simulink model "QD2_DroneStack_PID_2021a"  (R2026a)
settings: Solver=ode1  StopTime=inf  FixedStep=1/1000  EnableMultiTasking=on
InitFcn:
  | Motor_Mapping_7_Inch
model workspace (MAT data in the model file):
  target_system = 1
undefined symbols (not defined in the file): _Commander, _Stabilizer, datetime, HIL, KT, lf, log_, log_QD2_, m, Motor_Matrix, n, qc_get_step_size, s, saved_data
libraries: quarc_library x106, simulink x24, simulink_extras x3, sl_discontinuities x2
(part 2 of 5)

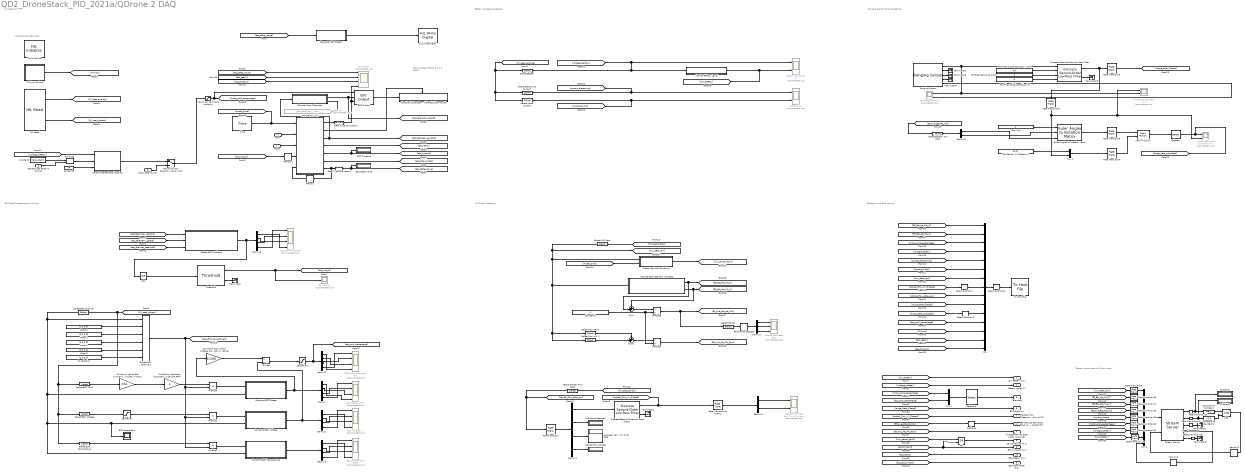
== system QD2_DroneStack_PID_2021a/QDrone 2 DAQ ==
  note: Battery Voltage Processing
  note: IMU Data Processing
  note: ESC Data Processing and Writing
  note: Initialize and read data
  note: Ranging Sensor Data Processing
  note: ESC Numbers
      |
      | FRONT
      | 3 1
      |
      | 2 0
      | BACK
  note: Blackbox and data routing
  note: HIL Read Write
  note: Stream drone data to Python class
  estop : Inport
  "Generalized Force (N, Nm) [4]" : Inport  Port=2
  Motor CMD (%) [4] : Inport  Port=3
  arm : Inport  Port=4
  AND : Logic  IconShape=distinctive  AllPortsSameDT=off  OutDataTypeStr=boolean
  Attitude Estimate from IMU Data : Subsystem
  Attitude Estimates (deg) : Scope  Commented=on  NumInputPorts=3
      settings: Title=Roll Estimates (deg)  ActiveDisplayYMinimum=-29.47666  ActiveDisplayYMaximum=31.43341  DataLoggingVariableName=ScopeData4
  "Average, Max, Min Pixel Rate" : Display
  Battery Monitoring (V) : Scope  Commented=on  NumInputPorts=2
      settings: Title=Battery Level (V)  ActiveDisplayYMinimum=16.17703  ActiveDisplayYMaximum=16.49829  DataLoggingVariableName=ScopeData2
  Choose Motor Telemetry : Subsystem
  Compare To Constant : simulink/Logic and Bit Operations/Compare To Constant  relop===  const=2  OutDataTypeStr=boolean
  Compare To Constant1 : simulink/Logic and Bit Operations/Compare To Constant  relop=>=  const=0  OutDataTypeStr=boolean
  Constant1 : Constant  Value=2
  Constant2 : Constant  Value=Motor_Matrix  OutDataTypeStr=double
  Constant3 : Constant  Value=KT  OutDataTypeStr=double
  Construct ESC Speed : Subsystem
  Construct ESC Temperature : Subsystem
  Construct ESC Voltage : Subsystem
  Convert to equivalent voltage (based on motor Kv rating) : Gain  Gain=1/1300
  Currents (A) : Scope  Commented=on  NumInputPorts=2
      settings: Title=Electronics Current (A)  ActiveDisplayYMinimum=0.11707  ActiveDisplayYMaximum=0.66845  DataLoggingVariableName=ScopeData3
  Data Type Conversion : DataTypeConversion  OutDataTypeStr=uint32  SaturateOnIntegerOverflow=off  RndMeth=Floor
  Data Type Conversion1 : DataTypeConversion  SaturateOnIntegerOverflow=off  RndMeth=Floor
  Demux{,1..3,8} (5 alike) : Demux
  Demux4 : Demux  Outputs=[2 1 3 1]
  Demux5 : Demux  Outputs=2
  Demux6 : Demux  Outputs=2
  Demux7 : Demux  Outputs=3
  Detect ESC Problems : Subsystem
  Discrete Second-Order Low-Pass Filter : quarc_library/Discrete/Discrete Second-Order Low-Pass Filter  params_source=External (input ports)  input_width=1  input_zeta=1  input_init=0  sample_time=qc_get_step_size*ceil(1/25/qc_get_step_size)
      settings: SourceProductName=QUARC Targets
  Discrete Second-Order Low-Pass Filter1 : quarc_library/Discrete/Discrete Second-Order Low-Pass Filter  params_source=Internal (dialog parameters)  input_width=1  input_zeta=1  input_init=0  sample_time=0.01
      settings: SourceProductName=QUARC Targets
  Display5 : Display
  Display6 : Display
  Divide : Product  Inputs=*/
  Divide by half of the number of poles in motor : Gain  Gain=2/14
  ESC Comm Problem : Scope  Commented=on  NumInputPorts=4
      settings: Title=Front Left (Motor 3)  ActiveDisplayYMinimum=-0.125  ActiveDisplayYMaximum=1.125  DataLoggingVariableName=ScopeData6
  ESC Motor Command (%) : Scope  Commented=on  NumInputPorts=4
      settings: Title=Front Left (Motor 3)  ActiveDisplayYMinimum=-0.00954  ActiveDisplayYMaximum=0.0859
  ESC Not OK : Scope  Commented=on
      settings: ActiveDisplayYMinimum=-0.125  ActiveDisplayYMaximum=1.125
  ESC Output : quarc_library/Data Acquisition/Generic/Transformations/ESC Output  protocol=DShot (raw)  sign=Unsigned
      settings: AttributesFormatString=%<protocol>  SourceProductName=QUARC Targets
  ESC Select Raw : Scope
      settings: ActiveDisplayYMinimum=-0.375  ActiveDisplayYMaximum=3.375  DataLoggingVariableName=ScopeData5
  ESC Speed (RPM) : Scope  Commented=on  NumInputPorts=4
      settings: Title=Front Left (Motor 3)  ActiveDisplayYMinimum=651.78571  ActiveDisplayYMaximum=1705.35714  DataLoggingVariableName=ScopeData4
  ESC State Value : Display
  ESC States : Scope  Commented=on  NumInputPorts=4
      settings: Title=ESC State  ActiveDisplayYMinimum=-11  ActiveDisplayYMaximum=99
  ESC Temperature (degC) : Scope  Commented=on  NumInputPorts=4
      settings: Title=Front Left (Motor 3)  ActiveDisplayYMinimum=-5.125  ActiveDisplayYMaximum=46.125  DataLoggingVariableName=ScopeData2
  ESC Timeout : Display
  ESC Voltage (V) : Scope  Commented=on  NumInputPorts=4
      settings: Title=Front Left (Motor 3)  ActiveDisplayYMinimum=-2.115  ActiveDisplayYMaximum=19.035  DataLoggingVariableName=ScopeData8
  Enabled Subsystem - Write ESC Commands : Subsystem  TreatAsAtomicUnit=on
  Euler Angles to Rotation Matrix : quarc_library/Math Operations/Matrices/Euler Angles to Rotation Matrix  menu_order=Relative Z-Y-X
      settings: SourceProductName=QUARC Targets
  Extract ESC Channels : MultiPortSwitch  DataPortOrder=Zero-based contiguous  Inputs=4  DataPortForDefault=Additional data port  zeroidx=on  SaturateOnIntegerOverflow=off  InputSameDT=off
  Force to percentage Mapping : MATLAB Function  TreatAsAtomicUnit=on
  Generate LED Pattern : Subsystem
  Goto19 : Goto  Commented=on  GotoTag=esc_telemetry_index
  HIL Initialize : quarc_library/Data Acquisition/Generic/Configuration/HIL Initialize  object_name=HIL-1  board_type=qdrone2  board_number=0  board_options=gyro0_fs=250;gyro0_rate=500;gyro0_bw=125;gyro0_ord=3;accel0_fs=16;accel0_rate=1000;accel0_bw=250;accel0_ord=3;temp0_bw=4000;gyro1_fs=250;gyro1_rate=500;gyro1_bw=125;gyro1_ord=3;accel1_fs=16;accel1_rate=1000;accel1_bw=400;accel1_ord=3;temp1_bw=4000;enc0_dir=0;enc1_dir=0;pwm03_dshot=1;opt_rate=121;  exclusive=off  active=on  hardware_clocks=[]  clock_modes=[]  initial_clock_frequencies=[]  set_clock_params_at_start=off  set_clock_params_at_switch_in=off  set_clock_frequencies_at_start=off  set_clock_frequencies_at_switch_in=off  analog_input_channels=[0:3]  analog_input_configurations=[]  analog_input_maximums=[3.3]  analog_input_minimums=[0]  set_analog_input_params_at_start=off  set_analog_input_params_at_switch_in=off  analog_output_channels=[]  analog_output_maximums=[]  analog_output_minimums=[]  initial_analog_outputs=[]  final_analog_outputs=[]  watchdog_analog_outputs=[]  set_analog_output_params_at_start=off  set_analog_output_params_at_switch_in=off  set_analog_outputs_at_start=off  set_analog_outputs_at_switch_in=off  set_analog_outputs_at_terminate=off  set_analog_outputs_at_switch_out=off  set_analog_outputs_on_watchdog=off  digital_input_channels=[0:5]  digital_output_channels=[6:11]  digital_output_configuration=[]  initial_digital_outputs=[0]  final_digital_outputs=[0]  watchdog_digital_outputs=[0 0 0 0 0 0]  set_digital_output_params_at_start=off  set_digital_output_params_at_switch_in=off  set_digital_outputs_at_start=on  set_digital_outputs_at_switch_in=off  set_digital_outputs_at_terminate=on  set_digital_outputs_at_switch_out=off  set_digital_outputs_on_watchdog=off  encoder_channels=[0:1]  quadrature=[4]  encoder_filter_frequency=100e6/1  initial_encoder_counts=[0]  set_encoder_params_at_start=on  set_encoder_params_at_switch_in=off  set_encoder_counts_at_start=on  set_encoder_counts_at_switch_in=off  pwm_channels=[0:5]  pwm_modes=[6 6 6 6 0]  pwm_frequency=[600000]  pwm_configuration=[0]  pwm_alignment=[0]  pwm_polarity=[1]  pwm_leading_deadband=[]  pwm_trailing_deadband=[]  initial_pwm_outputs=[0]  final_pwm_outputs=[0]  watchdog_pwm_outputs=[0]  set_pwm_params_at_start=on  set_pwm_params_at_switch_in=off  set_pwm_outputs_at_start=on  set_pwm_outputs_at_switch_in=off  set_pwm_outputs_at_terminate=on  set_pwm_outputs_at_switch_out=off  set_pwm_outputs_on_watchdog=on  other_output_channels=[]  initial_other_outputs=[]  final_other_outputs=[]  watchdog_other_outputs=[]  set_other_outputs_at_start=on  set_other_outputs_at_switch_in=off  set_other_outputs_at_terminate=on  set_other_outputs_at_switch_out=off  set_other_outputs_on_watchdog=off
  HIL Read : quarc_library/Data Acquisition/Generic/Immediate I//O/HIL Read  object_name=HIL-1  analog_channels=[3 1:2]  encoder_channels=[]  digital_channels=[]  other_channels=[3000:3002 4000:4002 3003:3005 4003:4005 17000:17006 17008:17009 17007 17010]  sample_time=qc_get_step_size  active=on  vector_output=on  port_labels=channel numbers  data_type_mode=Inherit via back propagation  encoder_data_type=double  digital_data_type=boolean
  HIL Write Digital : quarc_library/Data Acquisition/Generic/Immediate I//O/HIL Write Digital  object_name=HIL-1  channels=[6:11]  sample_time=-1  active=off  vector_input=on  port_labels=channel numbers
      settings: SourceProductName=QUARC Targets
  Height Estimate Compares (m) : Scope  Commented=on  NumInputPorts=2
      settings: Title=ToF Range Projected (m)  ActiveDisplayYMinimum=-0.10933  ActiveDisplayYMaximum=0.98394  DataLoggingVariableName=ScopeData3
  MATLAB Function : MATLAB Function  TreatAsAtomicUnit=on
  Manual Switch - Select Command Input : ManualSwitch
  Matrix Multiply : Product  Multiplication=Matrix(*)
  "Maximum Command Authority " : Saturate  UpperLimit=[1 1 1 1]  LowerLimit=[1 1 1 1]*0.025
  Memory : Memory
  Memory1 : Memory
  Memory2 : Memory  InheritSampleTime=on
  Memory3 : Memory  InheritSampleTime=on
  Monitor Battery Level : Subsystem
  Motor 0 : Constant  Value=[1 0 0 0]
  Motor 1 : Constant  Value=[0 1 0 0]
  Motor 2 : Constant  Value=[0 0 1 0]
  Motor 3 : Constant  Value=[0 0 0 1]
  Multiple by resolution (supposed to be 100 RPM) : Gain
  Mux : Mux  Inputs=15
  Mux1 : Mux  Inputs=2
  Mux2 : Mux  Inputs=2
  Mux3 : Mux  Inputs=9
  No selection : Constant  Value=[0 0 0 0]
  Number of Features : Display
  OR : Logic  Operator=OR  IconShape=distinctive  AllPortsSameDT=off  OutDataTypeStr=boolean
  OR1 : Logic  Operator=OR  Inputs=1  IconShape=distinctive  AllPortsSameDT=off  OutDataTypeStr=boolean
  Optical Flow Rate (Body Frame) (pixel/s) : Scope  Commented=on  NumInputPorts=2
      settings: Title=Body X Flow Rate (pixel/s)  ActiveDisplayYMinimum=-1312.1789  ActiveDisplayYMaximum=1008.97959
  Optical Flow Shutter : Display
  Product : Product
  Product1 : Product
  Product2 : Product
  Product3 : Product  Inputs=*/
  Product4 : Product  Inputs=*/
  Product5 : Product  Multiplication=Matrix(*)
  Radians to Degrees : simulink_extras/Transformations/Radians to Degrees
  Ranging Sensor : quarc_library/Devices/Third-Party/Sensors/Ranging Sensor  sensor_type=VL53L1X Time-of-flight  uri=i2c-cpu://localhost:0?address='0x29',baud='400000',memsize='512'  ranging_distance=Long  timing_budget=0.033  measurement_period=0.040  output_mode=Fixed-size output  samples_per_revolution=1300  max_distance=0.050  max_angle=5  sample_time=qc_get_step_size*ceil(1/25/qc_get_step_size)  show_versions=off  active=on
      settings: SourceProductName=QUARC Targets
  Rate Transition : RateTransition  OutPortSampleTime=0.01
  Rate Transition to 100Hz : RateTransition  OutPortSampleTime=0.01
  Rate Transition{1..2,7..12,14..20} (15 alike) : RateTransition
  Rate Transition3 : RateTransition  OutPortSampleTime=qc_get_step_size*ceil(1/25/qc_get_step_size)
  Rate Transition4 : RateTransition  OutPortSampleTime=qc_get_step_size*ceil(1/25/qc_get_step_size)
  Rate Transition5 : RateTransition  OutPortSampleTime=qc_get_step_size*ceil(1/25/qc_get_step_size)
  Rate Transition6 : RateTransition  OutPortSampleTime=qc_get_step_size
  Reshape : Reshape
  Saturation : Saturate  UpperLimit=17  LowerLimit=10
  Saturation1 : Saturate  UpperLimit=1  LowerLimit=0
  Select Battery : Selector  InputPortWidth=3  IndexOptions=Index vector (dialog)  Indices=[1]  OutputSizes=1
  Select ESC Channel : Selector  InputPortWidth=23  IndexOptions=Index vector (dialog)  Indices=[22]  OutputSizes=1
  Select ESC RPPM : Selector  InputPortWidth=23  IndexOptions=Index vector (dialog)  Indices=[20]  OutputSizes=1
  Select ESC Temperature : Selector  InputPortWidth=23  IndexOptions=Index vector (dialog)  Indices=[23]  OutputSizes=1
  Select ESC Voltage : Selector  InputPortWidth=23  IndexOptions=Index vector (dialog)  Indices=[21]  OutputSizes=1
  Select Electronics Current : Selector  InputPortWidth=3  IndexOptions=Index vector (dialog)  Indices=[2]  OutputSizes=1
  Select Est Att : Selector  InputPortWidth=9  IndexOptions=Index vector (dialog)  Indices=[1:3]  OutputSizes=1
  Select Est Roll and Pitch : Selector  InputPortWidth=9  IndexOptions=Index vector (dialog)  Indices=[1:2]  OutputSizes=1
  Select IMU Data : Selector  InputPortWidth=23  IndexOptions=Index vector (dialog)  Indices=[1:12]  OutputSizes=1
  Select Motor Current : Selector  InputPortWidth=3  IndexOptions=Index vector (dialog)  Indices=[3]  OutputSizes=1
  Select Optical Flow Data : Selector  InputPortWidth=23  IndexOptions=Index vector (dialog)  Indices=[13:19]  OutputSizes=1
  Select Raw IMU 0 : Selector  InputPortWidth=12  IndexOptions=Index vector (dialog)  Indices=[1:6]  OutputSizes=1
  Select Raw IMU 1 : Selector  InputPortWidth=12  IndexOptions=Index vector (dialog)  Indices=[7:12]  OutputSizes=1
  Selector : Selector  InputPortWidth=3  IndexOptions=Index vector (dialog)  Indices=[3]  OutputSizes=1
  Selector1 : Selector  InputPortWidth=8  IndexOptions=Index vector (dialog)  Indices=[4,8,3,7,2,6,1,5]  OutputSizes=1
  Sensor Failure Monitoring : Subsystem
  Stream Server : quarc_library/Communications/Basic/Stream Server  uri_source=Specify via dialog (do not evaluate)  uri=tcpip://localhost:18491?nagle='off'  send_buffer_size=1460  receive_buffer_size=1460  byte_order=little endian (Intel - LSB first)  optimization=Minimum latency  send_options=Send most recent data  receive_options=Receive most recent data  default_value=0  sample_time=qc_get_step_size*2  active=on  implementation=Use blocking I/O in a separate thread  send_fifo_size=1000  receive_fifo_size=1000  send_priority=0  receive_priority=0  send_dimensions=off  receive_dimensions=off  max_dimensions=-1  data_type=Inherited via back propagation  type_expr=BusObject
      settings: AttributesFormatString="\"tcpip://localhost:18491?nagle='off'\""
  Sum : Sum  Inputs=++|
  Sum1 : Sum  Inputs=++|
  Terminator{,1..7} (8 alike) : Terminator
  Threshold : quarc_library/Discontinuities/Threshold  operator=~=  param_src=Specify via dialog  threshold=0  duration=qc_get_step_size*300
      settings: SourceProductName=QUARC Targets
  Time : quarc_library/Sources/Time/Time  time_source=Wall clock  sample_time=qc_get_step_size
  Timing Monitors : Subsystem
  To Host File : quarc_library/Sinks/To Host/To Host File  source=Specify via dialog (do not evaluate)  file_name=saved_data\%m\log_QD2_%{regexprep(regexprep(char(datetime),':','-'),' ','_')}.mat  variable_name=QD2_data  decimation=1  sample_time=-1  file_format=MAT-file v.4  options=No header or footer  append=off  final_file_name=saved_data\\QD2_DroneStack_PID_2021a\\log_QD2_2026-09-08_13-10-08.mat  encoding=Default  bitrate=2000000
  ToF Filter Cutoff Frequency (rad) : Constant  Value=40
  ToF Filter Damping Ratio : Constant
  ToF Filter Initial Condition (m) : Constant  Value=0
  ToF Range Compare (m) : Scope  Commented=on  NumInputPorts=2
      settings: Title=ToF Range Filtered (m)  ActiveDisplayYMinimum=-0.12994  ActiveDisplayYMaximum=1.16949  DataLoggingVariableName=ScopeData2
  ToF Range Raw (m) : Scope  Commented=on  NumInputPorts=2
      settings: Title=ToF Range (m)  ActiveDisplayYMinimum=0.68027  ActiveDisplayYMaximum=0.99383
  ToF Sensor XY Offsets (m) : Constant  Value=[0 0]
  Zero Yaw : Constant  Value=0
  Low Battery (0,1) : Outport
  Battery Level (V) : Outport  Port=2
  Sensor Failure (0,1) : Outport  Port=3
  "Average BF IMU Data (rad/s, m/s/s) [6]" : Outport  Port=4
  Telemetry : Outport  Port=5
  BF Height (m) : Outport  Port=6
  Optical Flow Measurement (px/s) [2] : Outport  Port=7
  ESC Timeout (0,1) : Outport  Port=8
  ESC Stop Model (0,1) : Outport  Port=9
  ESC Ready (0,1) : Outport  Port=10
  "BF Attitude Estimates (rad, rad/s, rad/s/s) [9]" : Outport  Port=11
  wires:
  Force to percentage Mapping/1(Duty_Cycle) -> Manual Switch - Select Command Input/1
  Motor CMD (%) [4]/1 -> Manual Switch - Select Command Input/2
  "Generalized Force (N, Nm) [4]"/1 -> Product5/2
  [voltage_battery] -> Force to percentage Mapping/1(V_Bat_Act)
  Constant2/1 -> Product5/1
  Manual Switch - Select Command Input/1 -> "Maximum Command Authority "/1
  Constant3/1 -> Force to percentage Mapping/3(KT)
  Product5/1 -> Force to percentage Mapping/2(Motor_Forces)
  Reshape/1 -> "BF Attitude Estimates (rad, rad/s, rad/s/s) [9]"/1
  Saturation1/1 -> Demux2/1, [esc_cmd_percentage]
  [esc_stop_model] -> ESC Stop Model (0,1)/1
  [esc_ready] -> ESC Ready (0,1)/1
  [esc_timeout] -> ESC Timeout (0,1)/1, OR/2
  [BF_Ave_Att_IMU_Raw] -> "Average BF IMU Data (rad/s, m/s/s) [6]"/1
  [imu_sensor_fault] -> OR/1
  [BF_Ave_Est_Att_IMU] -> Reshape/1
  [optical_flow_XY_filtered] -> Optical Flow Measurement (px/s) [2]/1
  [range_data_filtered] -> BF Height (m)/1
  Selector1/1 -> Telemetry/1
  Mux2/1 -> Selector1/1
  [motor_cmd_percentage] -> Mux2/1
  [esc_cmd_percentage] -> Mux2/2
  [voltage_battery] -> Battery Level (V)/1
  [low_battery] -> Low Battery (0,1)/1
  [BF_Est_Att_IMU_1] -> Mux/2
  [voltage_battery] -> Mux/4
  [current_electronics] -> Mux/5
  [optical_flow_XY_filtered] -> Rate Transition7/1
  [esc_cmd_percentage] -> Mux/12
  [BF_Ave_Est_Att_IMU] -> Select Est Roll and Pitch/1
  [esc_ready] -> Mux/14
  [range_data_filtered] -> Mux/10
  Demux6/1 -> Euler Angles to Rotation Matrix/3
  Demux7/1 -> Attitude Estimates (deg)/1
  Ranging Sensor/5 -> ToF Range Raw (m)/2
  Discrete Second-Order Low-Pass Filter/2 -> Terminator5/1
  Radians to Degrees/1 -> Demux7/1
  Demux6/2 -> Euler Angles to Rotation Matrix/2
  Ranging Sensor/4 -> Terminator4/1
  Ranging Sensor/2 -> Terminator2/1
  ToF Filter Cutoff Frequency (rad)/1 -> Discrete Second-Order Low-Pass Filter/2
  ToF Sensor XY Offsets (m)/1 -> Mux1/1
  [Timing] -> Mux/13
  [current_motor] -> Mux/6
  Discrete Second-Order Low-Pass Filter1/1 -> Rate Transition to 100Hz/1, [optical_flow_XY_filtered]
  Demux7/2 -> Attitude Estimates (deg)/2
  Sensor Failure Monitoring/1(Sensor Fault) -> [imu_sensor_fault]
  [esc_state_value] -> Generate LED Pattern/1(ESC States)
  Select Est Att/1 -> Radians to Degrees/1
  Matrix Multiply/1 -> Selector/1
  Select Raw IMU 0/1 -> Sum1/1
  Select Raw IMU 1/1 -> Sum1/2
  [optical_flow_data_raw] -> Mux/9
  [esc_telemetry_select] -> Detect ESC Problems/2(ESC Channel Request [4])
  [esc_ready] -> ESC States/2
  Divide/1 -> Saturation1/1
  Select ESC Voltage/1 -> Saturation/1
  [motor_cmd_percentage] -> Mux/3
  Demux4/4 -> Optical Flow Shutter/1
  Monitor Battery Level/1(Low Battery) -> Battery Monitoring (V)/2, [low_battery]
  Demux3/1 -> ESC Temperature (degC)/4
  Convert to equivalent voltage (based on motor Kv rating)/1 -> Divide/1
  Demux4/2 -> Number of Features/1
  Rate Transition to 100Hz/1 -> Demux5/1
  Mux1/1 -> Rate Transition4/1
  Product3/1 -> [BF_Ave_Est_Att_IMU], Select Est Att/1
  Sum/1 -> Product3/1
  Demux4/1 -> Discrete Second-Order Low-Pass Filter1/1  "Optical Flow Pixel Rate (XY)"
  [imu_data_raw] -> Mux/7
  Demux5/2 -> Optical Flow Rate (Body Frame) (pixel/s)/2
  [esc_state_value] -> ESC States/1
  [hil_read_others] -> Select Optical Flow Data/1
  Discrete Second-Order Low-Pass Filter1/2 -> Terminator1/1
  Demux2/2 -> ESC Motor Command (%)/3
  estop/1 -> MATLAB Function/3(estop)
  Rate Transition4/1 -> Matrix Multiply/2
  Demux7/3 -> Attitude Estimates (deg)/3
  Sum1/1 -> Product4/1
  Threshold/2 -> Terminator/1
  [esc_channel_received] -> Detect ESC Problems/3(ESC Channel Reported [4])
  Generate LED Pattern/1(LED Command) -> HIL Write Digital/1
  Discrete Second-Order Low-Pass Filter/1 -> Rate Transition2/1, Rate Transition5/1
  Memory1/1 -> MATLAB Function/4(esc_problem)
  Demux4/3 -> "Average, Max, Min Pixel Rate"/1
  HIL Read/1 -> [hil_read_analog]
  Memory/1 -> MATLAB Function/5(pre_state)
  Product1/1 -> Construct ESC Voltage/1(ESC Data In [4])
  HIL Read/2 -> [hil_read_others]
  [esc_telemetry_enable] -> Detect ESC Problems/1(ESC Telemetry Enabled)
  Demux1/2 -> ESC Voltage (V)/3
  [model_time] -> Sensor Failure Monitoring/2(Model Time)
  Demux8/4 -> ESC Comm Problem/1
  Euler Angles to Rotation Matrix/1 -> Rate Transition3/1
  Select ESC Temperature/1 -> Product2/1
  MATLAB Function/6(stop_mdl) -> [esc_stop_model]
  Select Motor Current/1 -> Currents (A)/2, [current_motor]
  Construct ESC Voltage/1(ESC Data Out [4]) -> Demux1/1, Divide/2
  Demux1/1 -> ESC Voltage (V)/4
  Construct ESC Temperature/1(ESC Data Out [4]) -> Demux3/1
  Threshold/1 -> [esc_not_ok], ESC Not OK/1
  [esc_timeout] -> Mux/15
  MATLAB Function/4(esc_ready) -> [esc_ready]
  ToF Filter Initial Condition (m)/1 -> Discrete Second-Order Low-Pass Filter/4
  Ranging Sensor/1 -> Discrete Second-Order Low-Pass Filter/1, ToF Range Raw (m)/1, ToF Range Compare (m)/2
  MATLAB Function/2(cmd_enable) -> Enabled Subsystem - Write ESC Commands/Enable
  Ranging Sensor/3 -> Terminator3/1
  Select IMU Data/1 -> Select Raw IMU 1/1, Select Raw IMU 0/1, Attitude Estimate from IMU Data/1(IMU Data [12]), Sensor Failure Monitoring/1(IMU Data [12]), [imu_data_raw]
  No selection/1 -> Extract ESC Channels/6
  [BF_Est_Att_IMU_0] -> Mux/1
  [esc_timeout] -> ESC States/3
  OR1/1 -> Threshold/1
  [hil_read_analog] -> Select Battery/1, Select Motor Current/1, Select Electronics Current/1
  Demux8/2 -> ESC Comm Problem/3
  ToF Filter Damping Ratio/1 -> Discrete Second-Order Low-Pass Filter/3
  MATLAB Function/5(esc_timeout) -> ESC Timeout/1, [esc_timeout]
  Attitude Estimate from IMU Data/2("BF Estimated Attitude for IMU1 (rad, rad/s, rad/2^2) [9]") -> [BF_Est_Att_IMU_1], Sum/1
  Product/1 -> Construct ESC Speed/1(ESC Data In [4])
  [hil_read_others] -> Select IMU Data/1
  Rate Transition5/1 -> Mux1/2, Height Estimate Compares (m)/2, ToF Range Compare (m)/1
  "Maximum Command Authority "/1 -> ESC Output/1, [motor_cmd_percentage]
  Zero Yaw/1 -> Euler Angles to Rotation Matrix/1
  Data Type Conversion/1 -> ESC State Value/1, [esc_state_value]
  Demux1/3 -> ESC Voltage (V)/2
  Demux5/1 -> Optical Flow Rate (Body Frame) (pixel/s)/1
  Saturation/1 -> Product1/1
  Select Optical Flow Data/1 -> Rate Transition/1, [optical_flow_data_raw]
  Demux8/3 -> ESC Comm Problem/2
  Selector/1 -> Height Estimate Compares (m)/1, [range_data_projected]
  Attitude Estimate from IMU Data/1("BF Estimated Attitude for IMU0 (rad, rad/s, rad/2^2) [9]") -> [BF_Est_Att_IMU_0], Sum/2
  Rate Transition/1 -> Demux4/1
  Demux/3 -> ESC Speed (RPM)/2
  Detect ESC Problems/1(ESC Comm Problem [4]) -> Demux8/1, OR1/1
  Demux/4 -> ESC Speed (RPM)/1
  Motor 1/1 -> Extract ESC Channels/3
  Demux2/3 -> ESC Motor Command (%)/2
  Mux/1 -> Rate Transition6/1
  Demux/2 -> ESC Speed (RPM)/3
  Rate Transition3/1 -> Matrix Multiply/1
  Demux/1 -> ESC Speed (RPM)/4
  [esc_not_ok] -> Memory1/1
  Constant1/1 -> Product3/2, Product4/2
  Choose Motor Telemetry/2(Motor telemetry index) -> Goto19/1
  MATLAB Function/3(tele_enable) -> Choose Motor Telemetry/1(enable telemetry), [esc_telemetry_enable]
  [hil_read_others] -> Select ESC Channel/1, Select ESC Voltage/1, Select ESC Temperature/1, Select ESC RPPM/1
  Timing Monitors/1(Timings) -> [Timing]
  Motor 0/1 -> Extract ESC Channels/2
  Demux3/2 -> ESC Temperature (degC)/3
  Select Est Roll and Pitch/1 -> Demux6/1
  Motor 3/1 -> Extract ESC Channels/5
  Product4/1 -> [BF_Ave_Att_IMU_Raw]
  MATLAB Function/1(cmd) -> Data Type Conversion1/1
  Select ESC Channel/1 -> Construct ESC Speed/2(ESC Channel Select), Construct ESC Voltage/2(ESC Channel Select), ESC Select Raw/1, Construct ESC Temperature/2(ESC Channel Select), Extract ESC Channels/1
  Select Electronics Current/1 -> Currents (A)/1, [current_electronics]
  Multiple by resolution (supposed to be 100 RPM)/1 -> Product/1
  Rate Transition1/1 -> Mux/11
  Demux2/1 -> ESC Motor Command (%)/4
  Construct ESC Speed/1(ESC Data Out [4]) -> Convert to equivalent voltage (based on motor Kv rating)/1, Demux/1
  Motor 2/1 -> Extract ESC Channels/4
  Data Type Conversion1/1 -> ESC Output/3, ESC States/4
  MATLAB Function/7(state) -> Memory/1, Data Type Conversion/1
  Rate Transition2/1 -> [range_data_filtered]
  Choose Motor Telemetry/1(Motor telemetry select) -> ESC Output/2, [esc_telemetry_select]
  [range_data_projected] -> Rate Transition1/1
  Time/1 -> MATLAB Function/1(mdl_time), [model_time]
  Extract ESC Channels/1 -> Product2/2, Product1/2, Product/2, [esc_channel_received]
  Select Battery/1 -> Monitor Battery Level/1(Battery (V)), Battery Monitoring (V)/1, [voltage_battery]
  Divide by half of the number of poles in motor/1 -> Multiple by resolution (supposed to be 100 RPM)/1
  Demux1/4 -> ESC Voltage (V)/1
  Demux3/4 -> ESC Temperature (degC)/1
  Demux2/4 -> ESC Motor Command (%)/1
  arm/1 -> MATLAB Function/2(arm)
  ESC Output/1 -> Enabled Subsystem - Write ESC Commands/1(DShot Raw [4])
  Demux3/3 -> ESC Temperature (degC)/2
  Select ESC RPPM/1 -> Divide by half of the number of poles in motor/1
  Demux8/1 -> ESC Comm Problem/4
  Product2/1 -> Construct ESC Temperature/1(ESC Data In [4])
  OR/1 -> Sensor Failure (0,1)/1
  Rate Transition6/1 -> To Host File/1
  Rate Transition7/1 -> Mux/8
  Memory3/1 -> Stream Server/2
  Rate Transition9/1 -> Terminator7/1
  Rate Transition10/1 -> Mux3/6
  Stream Server/1 -> Rate Transition16/1
  Rate Transition17/1 -> Mux3/3
  Rate Transition11/1 -> Mux3/8
  Rate Transition12/1 -> Mux3/7
  [BF_Ave_Est_Att_IMU] -> Rate Transition19/1
  [BF_Est_Att_IMU_0] -> Rate Transition15/1
  AND/1 -> Memory3/1
  Rate Transition20/1 -> Mux3/5
  Rate Transition19/1 -> Mux3/4
  Stream Server/2 -> Rate Transition14/1
  Stream Server/4 -> Memory2/1
  Compare To Constant1/1 -> AND/2
  Memory2/1 -> Mux3/9
  [BF_Est_Att_IMU_1] -> Rate Transition17/1
  [low_battery] -> Rate Transition11/1
  Compare To Constant/1 -> AND/1
  [voltage_battery] -> Rate Transition12/1
  Rate Transition8/1 -> Mux3/1
  [motor_cmd_percentage] -> Rate Transition10/1
  Rate Transition15/1 -> Mux3/2
  [current_motor] -> Rate Transition20/1
  [imu_data_raw] -> Rate Transition8/1
  Stream Server/3 -> Rate Transition9/1
  Rate Transition14/1 -> Display6/1, Compare To Constant1/1
  Rate Transition18/1 -> Terminator6/1  "Connected (bool)"
  Rate Transition16/1 -> Display5/1, Compare To Constant/1
  Stream Server/5 -> Rate Transition18/1
  Mux3/1 -> Stream Server/1

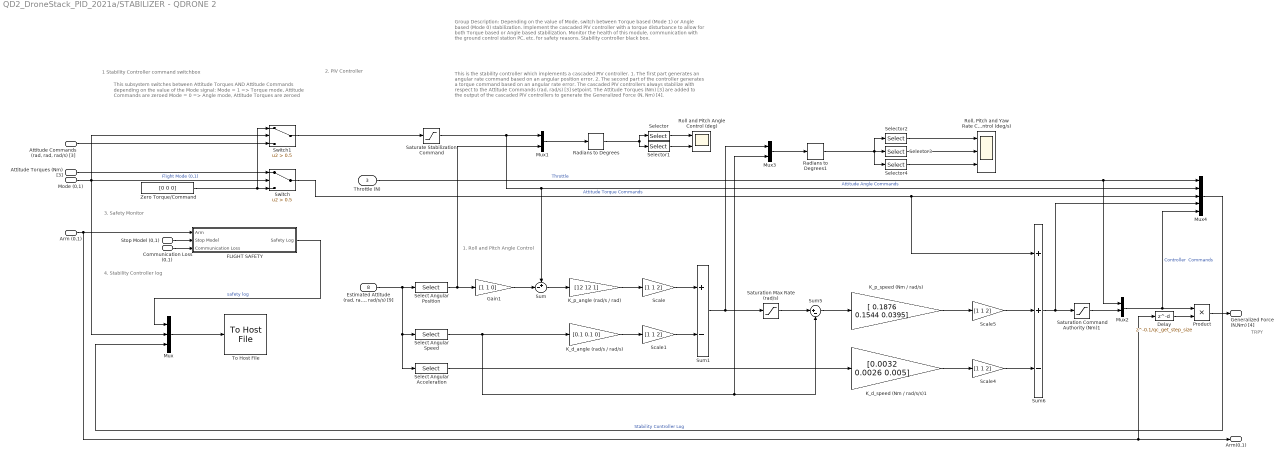
== system QD2_DroneStack_PID_2021a/STABILIZER - QDRONE 2 ==
  note: 3. Safety Monitor
  note: This subsystem switches between Attitude Torques AND Attitude Commands depending on
      | the value of the Mode signal:
      | Mode = 1	=> 		Torque mode, Attitude Commands are zeroed
      | Mode = 0	=> 		Angle mode, Attitude Torques are zeroed
  note: This is the stability controller which implements a cascaded PIV controller.
      | 1. The first part generates an angular rate command based on an angular position error.
      | 2. The second part of the controller generates a torque command based on an angular rate error.
      |
      | The cascaded PIV controllers always stabilize with respect to the Attitude Commands (rad, rad/s) [3] setpoint. The Attitude Torques (Nm) [3] are added to the output of the cascaded PIV controllers to generate the Generalized Force (N, Nm) [4].
  note: 1. Roll and Pitch Angle Control
  note: TRPY
  note: Group Description:
      |
      | Depending on the value of Mode, switch between Torque based (Mode 1) or Angle based (Mode 0) stabilization.
      | Implement the cascaded PIV controller with a torque disturbance to allow for both Torque based or Angle based stabilization.
      | Monitor the health of this module, communication with the ground control station PC, etc. for safety reasons.
      | Stability controller black box.
  note: 1 Stability Controller command switchbox
  note: 4. Stability Controller log
  note: 2. PIV Controller
  Mode (0,1) : Inport
  Stop Model (0,1) : Inport  Port=2
  Throttle (N) : Inport  Port=3
  Attitude Torques (Nm) [3] : Inport  Port=4
  "Attitude Commands (rad, rad, rad/s) [3]" : Inport  Port=5
  Arm (0,1) : Inport  Port=6
  Communication Loss (0,1) : Inport  Port=7
  "Estimated Attitude (rad, rad/s, rad/s/s) [9]" : Inport  Port=8
  Delay : Delay  DelayLength=0.1/qc_get_step_size
  FLIGHT SAFETY : Subsystem
  Gain1 : Gain  Gain=[1 1 0]
  K_d_angle (rad/s / rad/s) : Gain  Gain=[0.1 0.1 0]
  K_d_speed (Nm / rad/s/s)1 : Gain  Gain="[0.0032    0.0026     0.005]"
  K_p_angle (rad/s / rad) : Gain  Gain=[12 12 1]
  K_p_speed (Nm / rad/s) : Gain  Gain="[ 0.1876    0.1544    0.0395]"
  Mux : Mux  Inputs=3
  Mux1 : Mux  Inputs=2
  Mux2 : Mux  Inputs=2
  Mux3 : Mux  Inputs=2
  Mux4 : Mux  Inputs=5
  Product : Product
  Radians to Degrees : simulink_extras/Transformations/Radians to Degrees
  Radians to Degrees1 : simulink_extras/Transformations/Radians to Degrees
  Roll and Pitch Angle Control (deg) : Scope  NumInputPorts=2
      settings: Title=Roll (deg)  ActiveDisplayYMinimum=-2.00555  ActiveDisplayYMaximum=1.8629
  "Roll, Pitch and Yaw Rate Control (deg/s)" : Scope  NumInputPorts=3
      settings: ActiveDisplayYMinimum=-624.0016  ActiveDisplayYMaximum=680.10155  DataLoggingVariableName=ScopeData2
  Saturate Stabilization Command : Saturate  UpperLimit=[pi/4 pi/4 10*pi/18]  LowerLimit=[-pi/4 -pi/4 -10*pi/18]
  Saturation Command Authority (Nm)1 : Saturate  UpperLimit=[1.0915 0.8984 0.0984]  LowerLimit=-[1.0915 0.8984 0.0984]
  Saturation Max Rate (rad/s) : Saturate  UpperLimit=10*pi/3*[1 1 1]  LowerLimit=-10*pi/3*[1 1 1]
  Scale{,1,4..5} (4 alike) : Gain  Gain=[1 1 2]
  Select Angular Acceleration : Selector  InputPortWidth=9  IndexOptions=Index vector (dialog)  Indices=[7:9]  OutputSizes=1
  Select Angular Speed : Selector  InputPortWidth=9  IndexOptions=Index vector (dialog)  Indices=[4:6]  OutputSizes=1
  Select Angular Position : Selector  InputPortWidth=9  IndexOptions=Index vector (dialog)  Indices=[1:3]  OutputSizes=1
  Selector : Selector  InputPortWidth=6  IndexOptions=Index vector (dialog)  Indices=[1 4]  OutputSizes=1
  Selector1 : Selector  InputPortWidth=6  IndexOptions=Index vector (dialog)  Indices=[2 5]  OutputSizes=1
  Selector2 : Selector  InputPortWidth=6  IndexOptions=Index vector (dialog)  Indices=[1 4]  OutputSizes=1
  Selector3 : Selector  InputPortWidth=6  IndexOptions=Index vector (dialog)  Indices=[2 5]  OutputSizes=1
  Selector4 : Selector  InputPortWidth=6  IndexOptions=Index vector (dialog)  Indices=[3 6]  OutputSizes=1
  Sum : Sum  Inputs=+-|
  Sum1 : Sum  Inputs=+-
  Sum5 : Sum  Inputs=|+-
  Sum6 : Sum  Inputs=++-
  Switch : Switch  Criteria=u2 > Threshold  Threshold=0.5  SaturateOnIntegerOverflow=off  InputSameDT=off
  Switch1 : Switch  Criteria=u2 > Threshold  Threshold=0.5  SaturateOnIntegerOverflow=off  InputSameDT=off
  To Host File : quarc_library/Sinks/To Host/To Host File  source=Specify via dialog (do not evaluate)  file_name=saved_data/%m/log_%{regexprep(char(datetime),' ','_')}_Stabilizer.mat  variable_name=stabilizer_data  decimation=1  sample_time=-1  file_format=MAT-file v.5  options=No header or footer  append=off  final_file_name=saved_data/QD2_DroneStack_PID_2021a/log_2026-09-08_13-10-08_Stabilizer.mat  encoding=Default  bitrate=2000000
  Zero Torque/Command : Constant  Value=[0 0 0]
  Generalized Force (N,Nm) [4] : Outport  VectorParamsAs1DForOutWhenUnconnected=off
  Arm(0,1) : Outport  Port=2  VectorParamsAs1DForOutWhenUnconnected=off
  wires:
  Scale1/1 -> Sum1/2
  Scale/1 -> Sum1/1
  Delay/1 -> Product/2
  Zero Torque/Command/1 -> Switch1/1, Switch/3
  Attitude Torques (Nm) [3]/1 -> Switch/1
  "Attitude Commands (rad, rad, rad/s) [3]"/1 -> Switch1/3
  Radians to Degrees/1 -> Selector1/1, Selector/1
  K_d_angle (rad/s / rad/s)/1 -> Scale1/1
  Selector2/1 -> "Roll, Pitch and Yaw Rate Control (deg/s)"/1
  Selector/1 -> Roll and Pitch Angle Control (deg)/1
  Select Angular Speed/1 -> Mux3/2, Sum5/2, K_d_angle (rad/s / rad/s)/1
  K_p_angle (rad/s / rad)/1 -> Scale/1
  Selector4/1 -> "Roll, Pitch and Yaw Rate Control (deg/s)"/3
  Switch1/1 -> Saturate Stabilization Command/1
  Gain1/1 -> Sum/2
  Selector3/1 -> "Roll, Pitch and Yaw Rate Control (deg/s)"/2
  Mux1/1 -> Radians to Degrees/1
  "Estimated Attitude (rad, rad/s, rad/s/s) [9]"/1 -> Select Angular Speed/1, Select Angular Acceleration/1, Select Angular Position/1
  Radians to Degrees1/1 -> Selector3/1, Selector4/1, Selector2/1
  Switch/1 -> Sum6/1, Mux4/3  "Attitude Torque Commands"
  Selector1/1 -> Roll and Pitch Angle Control (deg)/2
  Throttle (N)/1 -> Mux4/1, Mux2/1  "Throttle"
  Select Angular Position/1 -> Mux1/2, Gain1/1
  Mux2/1 -> Product/1, Mux4/5  "Controller  Commands"
  Saturate Stabilization Command/1 -> Mux4/2, Sum/1, Mux1/1  "Attitude Angle Commands"
  Sum1/1 -> Mux3/1, Saturation Max Rate (rad/s)/1
  Mux3/1 -> Radians to Degrees1/1
  Arm (0,1)/1 -> FLIGHT SAFETY/1(Arm), Delay/1, Arm(0,1)/1
  Sum/1 -> K_p_angle (rad/s / rad)/1
  FLIGHT SAFETY/1(Safety Log) -> Mux/1  "safety log"
  Mode (0,1)/1 -> Mux/2, Switch1/2, Switch/2  "Flight Mode (0,1)"
  Mux4/1 -> Mux/3  "Stability Controller Log"
  Mux/1 -> To Host File/1
  Communication Loss (0,1)/1 -> FLIGHT SAFETY/3(Communication Loss)
  Stop Model (0,1)/1 -> FLIGHT SAFETY/2(Stop Model)
  Product/1 -> Generalized Force (N,Nm) [4]/1
  Saturation Max Rate (rad/s)/1 -> Sum5/1
  Sum5/1 -> K_p_speed (Nm / rad/s)/1
  K_p_speed (Nm / rad/s)/1 -> Scale5/1
  K_d_speed (Nm / rad/s/s)1/1 -> Scale4/1
  Scale4/1 -> Sum6/3
  Select Angular Acceleration/1 -> K_d_speed (Nm / rad/s/s)1/1
  Sum6/1 -> Mux4/4, Saturation Command Authority (Nm)1/1
  Saturation Command Authority (Nm)1/1 -> Mux2/2
  Scale5/1 -> Sum6/2

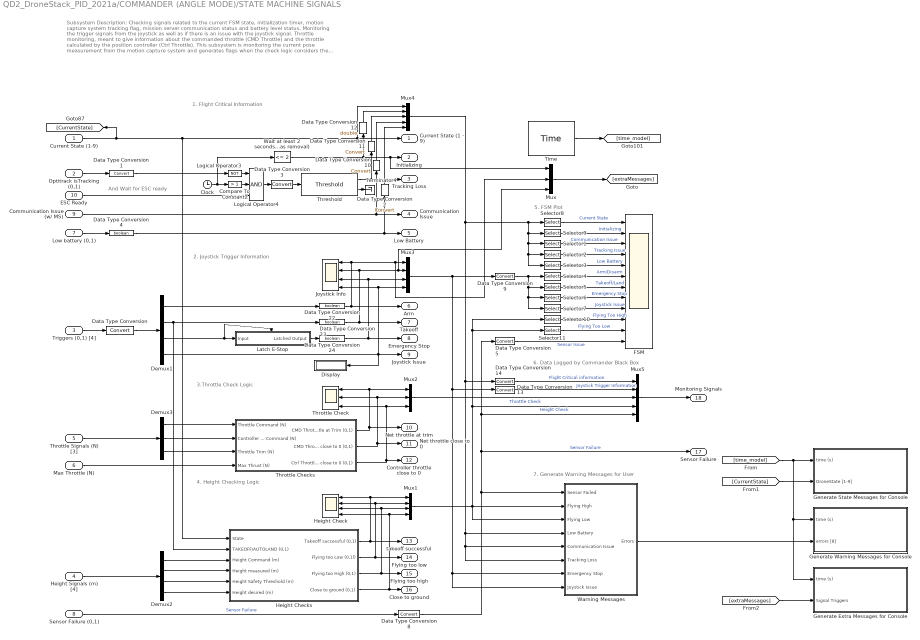
== system QD2_DroneStack_PID_2021a/COMMANDER (ANGLE MODE)/STATE MACHINE SIGNALS ==
  note: 4. Height Checking Logic
  note: 3.Throttle Check Logic
  note: 2. Joystick Trigger Information
  note: 1. Flight Critical Information
  note: 6. Data Logged by Commander Black Box
  note: 5. FSM Plot
  note: 7. Generate Warning Messages for User
  note: Subsystem Description:
      | Checking signals related to the current FSM state, initialization timer, motion capture system tracking flag, mission server communication status and battery level status.
      | Monitoring the trigger signals from the joystick as well as if there is an issue with the joystick signal.
      | Throttle monitoring, meant to give information about the commanded throttle (CMD Throttle) and the throttle calculated by the position controller (Ctrl Throttle).
      | This subsystem is monitoring the current pose measurement from the motion capture system and generates flags when the check logic considers the QDrone flying to close to ground, too high or too low as well as generate a successful take off flag.
      | A subset of the FSM monitoring signals are shown using this scope. These signals are what Quanser considers importnat for flight.
      | FSM signals sent to the blackbox for post flight monitoring.
      | Error message generation based on flags generated by the FSM signal checks.
  note: And Wait for ESC ready
  Current State (1-9) : Inport
  "Optitrack isTracking (0,1)  " : Inport  Port=2
  Triggers (0,1) [4] : Inport  Port=3
  Height Signals (m) [4] : Inport  Port=4
  Throttle Signals (N) [3] : Inport  Port=5
  "Max Throttle (N) " : Inport  Port=6
  Low battery (0,1) : Inport  Port=7
  Sensor Failure (0,1) : Inport  Port=8
  Communication Issue (w/ MS) : Inport  Port=9
  ESC Ready : Inport  Port=10
  Clock : Clock
  Compare To Constant2 : simulink/Logic and Bit Operations/Compare To Constant  relop=>  const=1  OutDataTypeStr=boolean
  Data Type Conversion{,1..3,5,8..11,13..14} (11 alike) : DataTypeConversion  SaturateOnIntegerOverflow=off  RndMeth=Floor
  Data Type Conversion12 : DataTypeConversion  OutDataTypeStr=double  SaturateOnIntegerOverflow=off  RndMeth=Floor
  Data Type Conversion{4,22..24} (4 alike) : DataTypeConversion  OutDataTypeStr=boolean  SaturateOnIntegerOverflow=off  RndMeth=Floor
  Demux1 : Demux  Outputs=[1 1 1 1]
  Demux2 : Demux
  Demux3 : Demux  Outputs=3
  Display : Display
  FSM : Scope  NumInputPorts=12
      settings: TimeSpan=30  Title=Current State  ActiveDisplayYMinimum=0.50000000000000011  ActiveDisplayYMaximum=5.5
  Generate Extra Messages for Console : Subsystem
  Generate State Messages for Console : Subsystem
  Generate Warning Messages for Console : Subsystem
  "Height Check " : Scope  NumInputPorts=4
      settings: Title=Takeoff Successful  ActiveDisplayYMinimum=-1  ActiveDisplayYMaximum=1  DataLoggingVariableName=ScopeData3
  Height Checks : Subsystem
  Joystick Info : Scope  NumInputPorts=4
      settings: Title=Arm
  Latch E-Stop : Subsystem  TreatAsAtomicUnit=on
  Logical Operator3 : Logic  Operator=NOT  AllPortsSameDT=off  OutDataTypeStr=boolean
  Logical Operator4 : Logic  Inputs=3  AllPortsSameDT=off  OutDataTypeStr=boolean
  Mux : Mux  Inputs=3
  Mux1 : Mux  Inputs=[1 1 1 1]
  Mux2 : Mux  Inputs=[1 1 1]
  Mux3 : Mux  Inputs=[1 1 1 1]
  Mux4 : Mux  Inputs=[1 1 1 1 1]
  Mux5 : Mux  Inputs=[5 4 3 4 1]
  Selector1 : Selector  InputPortWidth=5  IndexOptions=Index vector (dialog)  Indices=4  OutputSizes=1
  Selector10 : Selector  InputPortWidth=4  IndexOptions=Index vector (dialog)  Indices=3  OutputSizes=1
  Selector11 : Selector  InputPortWidth=4  IndexOptions=Index vector (dialog)  Indices=2  OutputSizes=1
  Selector2 : Selector  InputPortWidth=5  IndexOptions=Index vector (dialog)  Indices=3  OutputSizes=1
  Selector3 : Selector  InputPortWidth=5  IndexOptions=Index vector (dialog)  Indices=5  OutputSizes=1
  Selector4 : Selector  InputPortWidth=4  IndexOptions=Index vector (dialog)  Indices=1  OutputSizes=1
  Selector5 : Selector  InputPortWidth=4  IndexOptions=Index vector (dialog)  Indices=2  OutputSizes=1
  Selector6 : Selector  InputPortWidth=4  IndexOptions=Index vector (dialog)  Indices=3  OutputSizes=1
  Selector7 : Selector  InputPortWidth=4  IndexOptions=Index vector (dialog)  Indices=4  OutputSizes=1
  Selector8 : Selector  InputPortWidth=5  IndexOptions=Index vector (dialog)  Indices=1  OutputSizes=1
  Selector9 : Selector  InputPortWidth=5  IndexOptions=Index vector (dialog)  Indices=2  OutputSizes=1
  Terminator4 : Terminator
  Threshold : quarc_library/Discontinuities/Threshold  operator=>=  param_src=Specify via dialog  threshold=0.5  duration=0.2
      settings: SourceProductName=QUARC Targets
  Throttle Check : Scope  NumInputPorts=3
      settings: Title=Command Throttle At Trim  ActiveDisplayYMinimum=-0.125  ActiveDisplayYMaximum=1.125  DataLoggingVariableName=ScopeData2
  Throttle Checks : Subsystem
  Time : quarc_library/Sources/Time/Time  time_source=Wall clock  sample_time=qc_get_step_size
  "Wait at least 2 seconds to allow for initialization (e.g., bias removal)" : simulink/Logic and Bit Operations/Compare To Constant  relop=<=  const=2  OutDataTypeStr=boolean
  Warning Messages : Subsystem
  "Current State (1 - 9)  " : Outport  VectorParamsAs1DForOutWhenUnconnected=off
  Initializing : Outport  Port=2  VectorParamsAs1DForOutWhenUnconnected=off
  Tracking Loss : Outport  Port=3  VectorParamsAs1DForOutWhenUnconnected=off
  Communication Issue : Outport  Port=4  VectorParamsAs1DForOutWhenUnconnected=off
  Low Battery : Outport  Port=5  VectorParamsAs1DForOutWhenUnconnected=off
  Arm : Outport  Port=6  VectorParamsAs1DForOutWhenUnconnected=off
  Takeoff : Outport  Port=7  VectorParamsAs1DForOutWhenUnconnected=off
  Emergency Stop : Outport  Port=8  VectorParamsAs1DForOutWhenUnconnected=off
  "Joystick Issue " : Outport  Port=9  VectorParamsAs1DForOutWhenUnconnected=off
  Net throttle at trim : Outport  Port=10  VectorParamsAs1DForOutWhenUnconnected=off
  Net throttle close to 0 : Outport  Port=11  VectorParamsAs1DForOutWhenUnconnected=off
  Controller throttle close to 0 : Outport  Port=12  VectorParamsAs1DForOutWhenUnconnected=off
  takeoff successful : Outport  Port=13  VectorParamsAs1DForOutWhenUnconnected=off
  Flying too low : Outport  Port=14  VectorParamsAs1DForOutWhenUnconnected=off
  Flying too high : Outport  Port=15  VectorParamsAs1DForOutWhenUnconnected=off
  Close to ground : Outport  Port=16  VectorParamsAs1DForOutWhenUnconnected=off
  "  Sensor Failure" : Outport  Port=17  VectorParamsAs1DForOutWhenUnconnected=off
  Monitoring Signals : Outport  Port=18  VectorParamsAs1DForOutWhenUnconnected=off
  wires:
  ESC Ready/1 -> Logical Operator4/3
  [extraMessages] -> Generate Extra Messages for Console/2(Signal Triggers)
  Mux/1 -> [extraMessages]
  Warning Messages/1(Errors) -> Generate Warning Messages for Console/2(errors [8])
  [CurrentState] -> Generate State Messages for Console/2(DroneState [1-9])
  [time_model] -> Generate State Messages for Console/1(time (s)), Generate Extra Messages for Console/1(time (s)), Generate Warning Messages for Console/1(time (s))
  Time/1 -> [time_model]
  "Max Throttle (N) "/1 -> Throttle Checks/4(Max Thrust (N))
  "Wait at least 2 seconds to allow for initialization (e.g., bias removal)"/1 -> Initializing/1, Mux/1, Data Type Conversion12/1
  Data Type Conversion14/1 -> Mux5/1  "Flight Critical information"
  Data Type Conversion13/1 -> Mux5/2  "Joystick Trigger Information"
  Data Type Conversion12/1 -> Mux4/2
  Data Type Conversion11/1 -> Mux4/3
  Data Type Conversion10/1 -> Mux4/4
  Data Type Conversion2/1 -> Mux4/5
  Selector8/1 -> FSM/1  "Current State"
  Current State (1-9)/1 -> "Current State (1 - 9)  "/1, Mux4/1, Height Checks/1(State), [CurrentState]
  Data Type Conversion8/1 -> Warning Messages/1(Sensor Failed), Mux5/5, Data Type Conversion5/1, "  Sensor Failure"/1  "Sensor Failure"
  Data Type Conversion9/1 -> Selector6/1, Selector7/1, Selector5/1, Selector4/1
  Throttle Checks/3(Ctrl Throttle close to 0 (0,1)) -> Controller throttle close to 0/1, Throttle Check/3, Mux2/3
  Mux4/1 -> Selector8/1, Selector9/1, Selector1/1, Selector2/1, Selector3/1, Data Type Conversion14/1, Warning Messages/6(Tracking Loss), Warning Messages/5(Communication Issue), Warning Messages/4(Low Battery)
  Mux3/1 -> Data Type Conversion13/1, Warning Messages/8(Joystick Issue), Warning Messages/7("Emergency Stop "), Data Type Conversion9/1
  Mux2/1 -> Mux5/3  "Throttle Check"
  Mux1/1 -> Mux5/4, Selector10/1, Selector11/1, Warning Messages/2(Flying High), Warning Messages/3(Flying Low)  "Height Check"
  Mux5/1 -> Monitoring Signals/1
  Threshold/1 -> Tracking Loss/1, Data Type Conversion11/1
  Communication Issue (w/ MS)/1 -> Communication Issue/1, Data Type Conversion10/1
  Demux1/4 -> "Joystick Issue "/1, Mux3/4, Joystick Info/4, Display/1
  Data Type Conversion4/1 -> Low Battery/1, Data Type Conversion2/1
  Data Type Conversion22/1 -> Arm/1, Mux3/1, Mux/2, Joystick Info/1
  Data Type Conversion23/1 -> Takeoff/1, Mux3/2, Mux/3, Joystick Info/2
  Data Type Conversion24/1 -> Emergency Stop/1, Mux3/3, Joystick Info/3
  Selector11/1 -> FSM/11  "Flying Too Low"
  Selector10/1 -> FSM/10  "Flying Too High"
  Data Type Conversion5/1 -> FSM/12  "Sensor Issue"
  Selector7/1 -> FSM/9  "Joystick Issue"
  Selector6/1 -> FSM/8  "Emergency Stop"
  Selector5/1 -> FSM/7  "Takeoff/Land"
  Selector4/1 -> FSM/6  "Arm/Disarm"
  Selector3/1 -> FSM/5  "Low Battery"
  Selector2/1 -> FSM/4  "Tracking Issue"
  Selector1/1 -> FSM/3  "Communication Issue"
  Selector9/1 -> FSM/2  "Initializing"
  Demux1/3 -> Latch E-Stop/Trigger, Latch E-Stop/1(Input)
  Latch E-Stop/1(Latched Output) -> Data Type Conversion24/1
  "Optitrack isTracking (0,1)  "/1 -> Data Type Conversion1/1
  Logical Operator3/1 -> Logical Operator4/1
  Threshold/2 -> Terminator4/1
  Logical Operator4/1 -> Data Type Conversion3/1
  Clock/1 -> Compare To Constant2/1, "Wait at least 2 seconds to allow for initialization (e.g., bias removal)"/1
  Compare To Constant2/1 -> Logical Operator4/2
  Data Type Conversion3/1 -> Threshold/1
  Data Type Conversion1/1 -> Logical Operator3/1
  Sensor Failure (0,1)/1 -> Data Type Conversion8/1  "Sensor Failure"
  Height Checks/2(Flying too Low (0,1l)) -> "Height Check "/2, Mux1/2, Flying too low/1
  Low battery (0,1)/1 -> Data Type Conversion4/1
  Data Type Conversion/1 -> Demux1/1
  Height Checks/4(Close to ground (0,1)) -> Close to ground/1, Mux1/4, "Height Check "/4
  Height Checks/3(Flying too High (0,1)) -> Flying too high/1, "Height Check "/3, Mux1/3
  Throttle Checks/1(CMD Throttle at Trim (0,1)) -> Throttle Check/1, Mux2/1, Net throttle at trim/1
  Demux3/3 -> Throttle Checks/3(Throttle Trim (N))
  Demux3/2 -> Throttle Checks/2(Controller Throttle Command (N))
  Demux2/2 -> Height Checks/4(Height measured (m))
  Demux1/2 -> Height Checks/2(TAKEOFF/AUTOLAND (0,1)), Data Type Conversion23/1
  Demux2/3 -> Height Checks/5(Height Safety Threshold (m))
  Height Checks/1(Takeoff successful (0,1)) -> Mux1/1, "Height Check "/1, takeoff successful/1
  Throttle Checks/2(CMD Throttle close to 0 (0,1)) -> Net throttle close to 0/1, Throttle Check/2, Mux2/2
  Demux1/1 -> Data Type Conversion22/1
  Throttle Signals (N) [3]/1 -> Demux3/1
  Demux2/4 -> Height Checks/6(Height desired (m))
  Height Signals (m) [4]/1 -> Demux2/1
  Demux3/1 -> Throttle Checks/1(Throttle Command (N))
  Demux2/1 -> Height Checks/3(Height Command (m))
  Triggers (0,1) [4]/1 -> Data Type Conversion/1

== system QD2_DroneStack_PID_2021a/COMMANDER (ANGLE MODE)/Signal Smoothing ==
  "High Frequency Controller Commands (N,rad, rad/s)[4]" : Inport
  Constant4 : Constant
  Constant5 : Constant  Value=100
  Mux : Mux  Inputs=2
  Second-Order Low-Pass Filter : quarc_library/Continuous/Second-Order Low-Pass Filter  params_source=External (input ports)  input_width=60  input_zeta=1  input_init=0
  Selector1 : Selector  InputPortWidth=4  IndexOptions=Index vector (dialog)  Indices=[3:4]  OutputSizes=1
  Selector3 : Selector  InputPortWidth=4  IndexOptions=Index vector (dialog)  Indices=[1:2]  OutputSizes=1
  Terminator : Terminator
  "Smoothed Controller Commands (N,rad, rad/s)[4]" : Outport
  wires:
  Second-Order Low-Pass Filter/2 -> Terminator/1
  Constant5/1 -> Second-Order Low-Pass Filter/2
  Constant4/1 -> Second-Order Low-Pass Filter/3
  Selector3/1 -> Second-Order Low-Pass Filter/1, Second-Order Low-Pass Filter/4
  Second-Order Low-Pass Filter/1 -> Mux/1
  Selector1/1 -> Mux/2
  Mux/1 -> "Smoothed Controller Commands (N,rad, rad/s)[4]"/1
  "High Frequency Controller Commands (N,rad, rad/s)[4]"/1 -> Selector3/1, Selector1/1
